simulink model "Extended_model"  (R2021b)
settings: Solver=ode45  StartTime=0.0  StopTime=10.0  RelTol=1e-3  EnableMultiTasking=on
values from neighbouring files (symbols this model uses):
  Ask = [0 1 0 0 ... (first row only)    [H_inf_ctrl.m]    (also in H_inf_ctrl_11_2.m; H_inf_ctrl_11_2_m.m)
  Bsk = [0 0 0 0 ... (first row only)    [H_inf_ctrl.m]    (also in H_inf_ctrl_11_2.m; H_inf_ctrl_11_2_m.m)
  Csk = [0 1 0 0 ... (first row only)    [H_inf_ctrl.m]    (also in H_inf_ctrl_11_2.m; H_inf_ctrl_11_2_m.m)
  Dsk = zeros(2,4)    [H_inf_ctrl.m]    (also in H_inf_ctrl_11_2.m; H_inf_ctrl_11_2_m.m)
libraries: cstblocks x4
settings Model: Creator=Alireza  LastModifiedBy=rivaa
settings SolverCC: AlgebraicLoopSolver=TrustRegion
settings DataIOCC: LimitDataPoints=on  SaveFormat=Array  SignalLoggingSaveFormat=ModelDataLogs  ReturnWorkspaceOutputs=off
settings OptimizationCC: ExpressionDepthLimit=2147483647  LifeSpan=inf
settings DebuggingCC: UnderspecifiedInitializationDetection=Classic  MergeDetectMultiDrivingBlocksExec=none  SolverPrmCheckMsg=warning  FcnCallInpInsideContextMsg=warning  StateNameClashWarn=warning  SFUnexpectedBacktrackingDiag=warning  SFNoUnconditionalDefaultTransitionDiag=warning  SFExecutionAtInitializationDiag=none  SFMachineParentedDataDiag=warning  ArithmeticOperatorsInVariantConditions=warning
settings HardwareCC: ProdBitPerPointer=32  ProdBitPerSizeT=32  ProdBitPerPtrDiffT=32  ProdLargestAtomicFloat=None  ProdIntDivRoundTo=Undefined  ProdEndianess=Unspecified  ProdWordSize=32  ProdHWDeviceType=32-bit Generic
settings ModelReferenceCC: PropagateSignalLabelsOutOfModel=off
settings SFSimCC: SimUseLocalCustomCode=off  CustomCodeUndefinedFunction=UseInterfaceOnly
settings RTWCC: RTWUseLocalCustomCode=off
settings CodeAppCC: StateflowObjectComments=on
settings GRTTargetCC: TargetLangStandard=C89/C90 (ANSI)  CombineOutputUpdateFcns=off  GRTInterface=on
settings ConfigComp: CovMetricSettings=dw  CovSaveCumulativeToWorkspaceVar=on  CovSaveSingleToWorkspaceVar=on  CovExternalEMLEnable=off

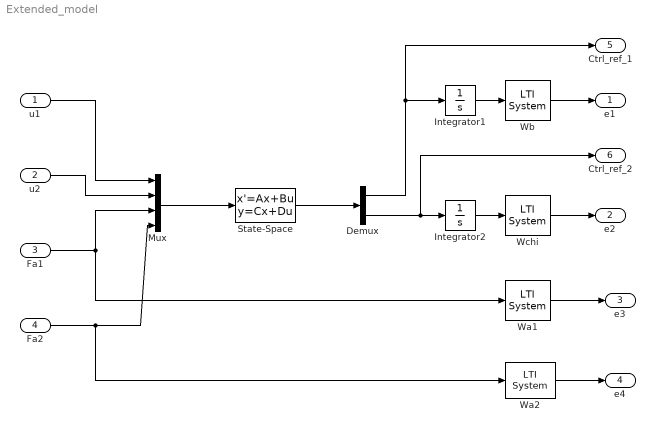
== system Extended_model ==
  u1 : Inport
  u2 : Inport  Port=2
  Fa1 : Inport  Port=3
  Fa2 : Inport  Port=4
  Demux : Demux  Outputs=2
  Integrator1 : Integrator
  Integrator2 : Integrator
  Mux : Mux
  State-Space : StateSpace  A=Ask  B=Bsk  C=Csk  D=Dsk  InitialCondition=0
  Wa1 : cstblocks/LTI System  sys=Wa1  IC=[]
  Wa2 : cstblocks/LTI System  sys=Wa2  IC=[]
  Wb : cstblocks/LTI System  sys=Wb  IC=[]
  Wchi : cstblocks/LTI System  sys=Wchi  IC=[]
  e1 : Outport
  e2 : Outport  Port=2
  e3 : Outport  Port=3
  e4 : Outport  Port=4
  Ctrl_ref_1 : Outport  Port=5
  Ctrl_ref_2 : Outport  Port=6
  wires:
  u1/1 -> Mux/1
  u2/1 -> Mux/2
  Fa1/1 -> Mux/3, Wa1/1
  Fa2/1 -> Mux/4, Wa2/1
  Wa1/1 -> e3/1
  Wa2/1 -> e4/1
  Mux/1 -> State-Space/1
  State-Space/1 -> Demux/1
  Demux/1 -> Ctrl_ref_1/1, Integrator1/1
  Demux/2 -> Ctrl_ref_2/1, Integrator2/1
  Wb/1 -> e1/1
  Wchi/1 -> e2/1
  Integrator1/1 -> Wb/1
  Integrator2/1 -> Wchi/1
